simulink model "ode_engine_sim"  (R2022a)
settings: Solver=VariableStepAuto  StartTime=0.0  StopTime=1  MinStep=1e-3
model workspace (MAT data in the model file):
  A_inj = 0.0001076
  C_d = 0.7
  L_grain = 0.6
  PCrit = 72.51
  TCrit = 309.57
  ThermoModel.kin.owner = 1
  ThermoModel.kin.id = 3
  ThermoModel.th.owner = 1
  ThermoModel.th.tp_id = 3
  ThermoModel.tr.id = 3
  ThermoModel.tr.th.owner = 1
  ThermoModel.tr.th.tp_id = 3
  ThermoModel.ThermoPhase.owner = 1
  ThermoModel.ThermoPhase.tp_id = 3
  ThermoModel.Kinetics.owner = 1
  ThermoModel.Kinetics.id = 3
  ThermoModel.Transport.id = 3
  ThermoModel.Transport.th.owner = 1
  ThermoModel.Transport.th.tp_id = 3
  V_tank = 0.0235
  a = 0.397
  inital_cc_pressure = 101325
  inital_run_tank_temperature = 293.3
  m_reg = 1
  n = 0.367
  r_initial = 50
  rhoCrit = 452
  rho_f = 1100
  throat_diam = 0.039385
settings Model: Creator=Artem Sotnikov  LastModifiedBy=Artem Sotnikov
settings SolverCC: MaxConsecutiveMinStep=auto  ShapePreserveControl=EnableAll  ZeroCrossControl=EnableAll  ZeroCrossAlgorithm=Adaptive  EnableFixedStepZeroCrossing=on

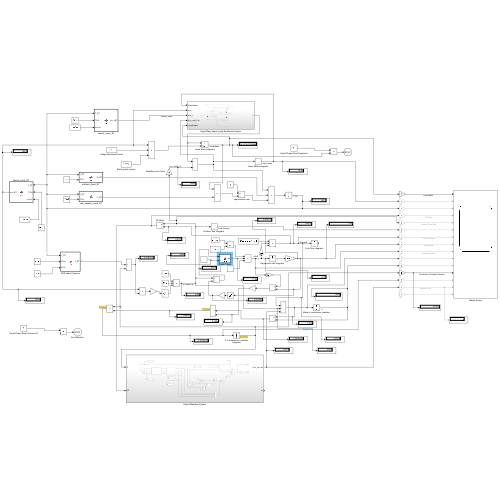
[thumbnail: Simulink's stored preview of the top-level diagram]
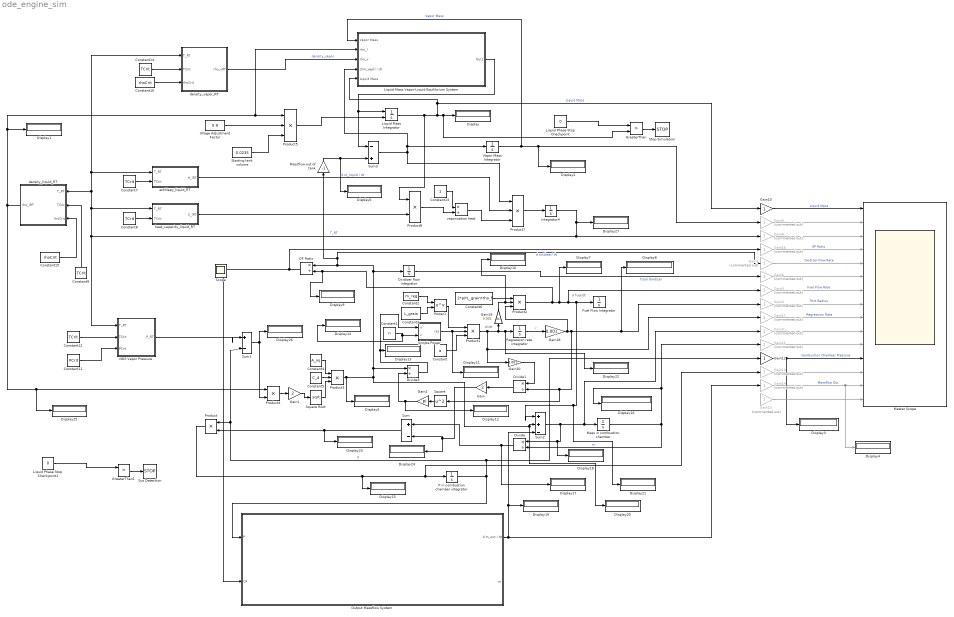
== system ode_engine_sim ==
  note: d fuel/dt
  note: dr/dt
  Constant : Constant  Value=a
  Constant1 : Constant  Value=n
  Constant10 : Constant  Value=rhoCrit
  Constant11 : Constant  Value=PCrit
  Constant{7..9,12,14} (5 alike) : Constant  Value=TCrit
  Constant13 : Constant
  Constant15 : Constant  Value=rhoCrit
  Constant2 : Constant  Value=m_reg
  Constant3 : Constant  Value=L_grain
  Constant4 : Constant  Value=A_inj
  Constant5 : Constant  Value=C_d
  Constant6 : Constant  Value=2*pi*L_grain*rho_f
  Display{,1..27} (28 alike) : Display
  Divide : Product  Inputs=*/
  Divide1 : Product  Inputs=*/
  Divide3 : Product  Inputs=*/
  Fuel Flow Intagrator : Integrator  InitialCondition=1e-6
  Gain : Gain  Gain=2
  Gain1 : Gain  Gain=2
  Gain10 : Gain
  Gain{3..9,11,13..17} (13 alike) : Gain  Commented=on
  Gain12 : Gain
  Gain18 : Gain  Gain=0.001
  Gain19 : Gain  Gain=0.001
  Gain2 : Gain  Gain=pi
  Gain20 : Gain  Gain=0.001
  GreaterThan : RelationalOperator  Operator=>  OutDataTypeStr=boolean  RndMeth=Simplest  InputSameDT=off
  GreaterThan1 : RelationalOperator  Operator=>  OutDataTypeStr=boolean  RndMeth=Simplest  InputSameDT=off
  Integrator4 : Integrator  InitialCondition=inital_run_tank_temperature
  Liquid Mass Integrator : Integrator  InitialConditionSource=external
  Liquid Mass Vapor-Liquid Equilibrium System : Subsystem
  Liquid Phase Stop Checkpoint : Constant  Value=0
  Liquid Phase Stop Checkpoint1 : Constant  Value=0
  Mass in combustion chamber : Integrator  InitialCondition=1e-9
  Massflow out of tank : Gain  Gain=-1
  Master Scope : Scope  NumInputPorts=15
  NOS Vapor Pressure : MATLAB Function  TreatAsAtomicUnit=on
  OF Ratio : Product  Inputs=*/
  Output Massflow System : Subsystem
  Oxidizer flow integrator : Integrator  InitialCondition=1e-6
  P in combustion chamber integrator : Integrator  InitialCondition=inital_cc_pressure  ZeroCross=off
  Power1 : Math  Operator=pow
  Product : Product
  Product{1..3,5,7} (5 alike) : Product  Inputs=3
  Product4 : Product
  Product8 : Product
  Regression rate integrator : Integrator  InitialCondition=r_initial
  Simple Power : MATLAB Function  TreatAsAtomicUnit=on
  Square : Math  Operator=square
  Square Root : Sqrt
  Starting tank volume : Constant  Value=0.0235
  Stop Simulation : Stop
  Sum : Sum  Inputs=|+-  RndMeth=Round
  Sum1 : Sum  Inputs=|+-
  Sum2 : Sum  Inputs=|++-
  Sum3 : Sum  Inputs=-+
  Sus Detection : Stop
  Ullage Adjustment Factor : Constant  Value=0.9
  Vapor Mass Integrator : Integrator  InitialCondition=1e-6
  "density_liquid_RT " : MATLAB Function  TreatAsAtomicUnit=on
  density_vapor_RT : MATLAB Function  TreatAsAtomicUnit=on
  enthlapy_liquid_RT : MATLAB Function  TreatAsAtomicUnit=on
  heat_capacity_liquid_RT : MATLAB Function  TreatAsAtomicUnit=on
  vaporization heat : Product  Inputs=*/
  Scope : Scope
  wires:
  P in combustion chamber integrator/1 -> Gain12/1, Product/1, Sum1/2, Output Massflow System/1(P)  "P"
  Sum/1 -> Display23/1, Product/2
  Mass in combustion chamber/1 -> Display16/1, Gain11/1, Divide/2  "m"
  Product/1 -> Display15/1, Gain13/1, P in combustion chamber integrator/1
  Product1/1 -> Display22/1, Regression rate integrator/1, Gain19/1, Gain17/1, Gain20/1
  Regression rate integrator/1 -> Gain18/1  "r"
  Divide1/1 -> Gain/1
  Power1/1 -> Product1/1
  Constant/1 -> Product1/3
  Constant1/1 -> Simple Power/2(v), Display14/1
  Constant2/1 -> Power1/1
  Constant3/1 -> Power1/2
  Constant5/1 -> Product3/2
  Constant4/1 -> Product3/1
  Square Root/1 -> Product3/3
  Product3/1 -> Display5/1, Display20/1, Sum2/2, Massflow out of tank/1, Gain7/1, OF Ratio/1, Oxidizer flow integrator/1, Divide3/1  "d oxidizer/ dt"
  Gain1/1 -> Square Root/1
  NOS Vapor Pressure/1(P_RT) -> Sum1/1
  Product4/1 -> Gain1/1
  Sum1/1 -> Product4/2, Display26/1
  "density_liquid_RT "/1(rho_lRT) -> Display1/1, Product5/1, Liquid Mass Vapor-Liquid Equilibrium System/2(rho_l), Display25/1, Product4/1
  Square/1 -> Gain2/1
  Gain2/1 -> Display12/1, Divide3/2
  Product2/1 -> Display9/1, OF Ratio/2, Display7/1, Display21/1, Sum2/1, Fuel Flow Intagrator/1, Gain5/1
  Constant6/1 -> Product2/1
  Integrator4/1 -> Display27/1, NOS Vapor Pressure/1(T_RT), enthlapy_liquid_RT/1(T_RT), density_vapor_RT/1(T_RT), "density_liquid_RT "/1(T_RT), heat_capacity_liquid_RT/1(T_RT), Gain8/1  "T_RT"
  Product7/1 -> Integrator4/1
  enthlapy_liquid_RT/1(H_lRT) -> Product7/2
  Constant13/1 -> vaporization heat/1
  Product8/1 -> vaporization heat/2
  heat_capacity_liquid_RT/1(C_lRT) -> Product8/2
  vaporization heat/1 -> Product7/3
  Massflow out of tank/1 -> Display6/1, Sum3/2  "d m_liquid / dt"
  Sum3/1 -> Vapor Mass Integrator/1, Liquid Mass Vapor-Liquid Equilibrium System/4(d(m_vapl) / dt), Product7/1
  Vapor Mass Integrator/1 -> Liquid Mass Vapor-Liquid Equilibrium System/1(Vapor Mass), Display2/1, Gain9/1  "Vapor Mass"
  OF Ratio/1 -> Gain16/1, Output Massflow System/2(OF)
  Output Massflow System/1(d m_out / dt) -> Display19/1, Sum2/3, Gain14/1
  Liquid Mass Vapor-Liquid Equilibrium System/1(Out1) -> Sum3/1, Liquid Mass Integrator/1
  Liquid Mass Integrator/1 -> Product8/1, Display/1, GreaterThan/2, Liquid Mass Vapor-Liquid Equilibrium System/5(Liquid Mass), Gain10/1  "Liquid Mass"
  Oxidizer flow integrator/1 -> Gain6/1  "Total Oxidizer"
  Gain3/1 -> Master Scope/10
  Gain11/1 -> Master Scope/11
  Gain4/1 -> Master Scope/8  "Port Radius"
  Gain5/1 -> Master Scope/7  "Fuel Flow Rate"
  Gain7/1 -> Master Scope/5  "Oxidizer Flow Rate"
  Gain8/1 -> Master Scope/3
  Gain9/1 -> Master Scope/2
  Gain10/1 -> Master Scope/1  "Liquid Mass"
  Gain12/1 -> Display3/1, Master Scope/12  "Combustion Chamber Pressure"
  Gain13/1 -> Master Scope/13
  Gain14/1 -> Display4/1, Master Scope/14  "Massflow Out"
  Gain15/1 -> Master Scope/15
  Gain16/1 -> Master Scope/4  "OF Ratio"
  Gain17/1 -> Master Scope/9  "Regression Rate"
  density_vapor_RT/1(rho_vRT) -> Liquid Mass Vapor-Liquid Equilibrium System/3(rho_v)  "density_vapor"
  Constant7/1 -> enthlapy_liquid_RT/2(TCrit)
  Constant8/1 -> heat_capacity_liquid_RT/2(TCrit)
  Constant9/1 -> "density_liquid_RT "/2(TCrit)
  Constant10/1 -> density_vapor_RT/3(rhoCrit)
  Constant11/1 -> NOS Vapor Pressure/3(PCrit)
  Constant12/1 -> NOS Vapor Pressure/2(TCrit)
  Constant14/1 -> density_vapor_RT/2(TCrit)
  Constant15/1 -> "density_liquid_RT "/3(rhoCrit)
  Gain6/1 -> Master Scope/6
  Starting tank volume/1 -> Product5/3
  Product5/1 -> Liquid Mass Integrator/2
  Ullage Adjustment Factor/1 -> Product5/2
  GreaterThan/1 -> Stop Simulation/1
  Liquid Phase Stop Checkpoint/1 -> GreaterThan/1
  Divide/1 -> Display17/1, Sum/1
  Gain/1 -> Display24/1, Sum/2
  Gain18/1 -> Divide1/2, Square/1, Display8/1, Gain4/1, Product2/3
  Divide3/1 -> Simple Power/1(u), Display13/1
  Simple Power/1(res) -> Display11/1, Product1/2
  Gain19/1 -> Display10/1, Product2/2
  Gain20/1 -> Divide1/1
  Sum2/1 -> Gain3/1, Mass in combustion chamber/1, Display18/1, Divide/1
  Liquid Phase Stop Checkpoint1/1 -> GreaterThan1/1
  GreaterThan1/1 -> Sus Detection/1

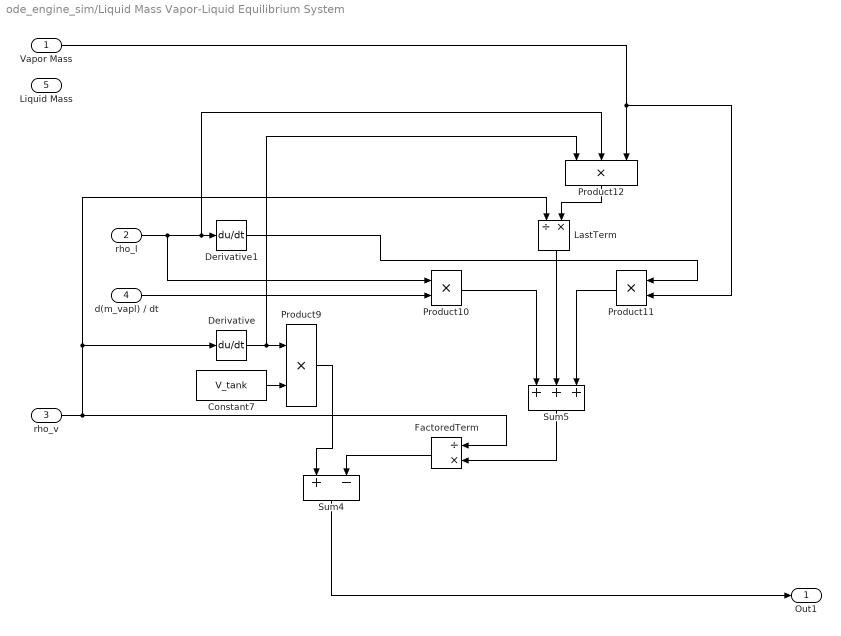
== system ode_engine_sim/Liquid Mass Vapor-Liquid Equilibrium System ==
  Vapor Mass : Inport
  rho_l : Inport  Port=2
  rho_v : Inport  Port=3
  d(m_vapl) / dt : Inport  Port=4
  Liquid Mass : Inport  Port=5
  Constant7 : Constant  Value=V_tank
  Derivative : Derivative
  Derivative1 : Derivative
  FactoredTerm : Product  Inputs=/*
  LastTerm : Product  Inputs=/*
  Product10 : Product
  Product11 : Product
  Product12 : Product  Inputs=3
  Product9 : Product
  Sum4 : Sum  Inputs=+-
  Sum5 : Sum  Inputs=+++
  Out1 : Outport
  wires:
  Product9/1 -> Sum4/1
  Derivative/1 -> Product9/1, Product12/1
  rho_v/1 -> Derivative/1, LastTerm/1, FactoredTerm/1
  Product10/1 -> Sum5/1
  Derivative1/1 -> Product11/1
  LastTerm/1 -> Sum5/2
  Product11/1 -> Sum5/3
  rho_l/1 -> Product10/1, Product12/2, Derivative1/1
  Product12/1 -> LastTerm/2
  Sum5/1 -> FactoredTerm/2
  Constant7/1 -> Product9/2
  FactoredTerm/1 -> Sum4/2
  Sum4/1 -> Out1/1
  d(m_vapl) / dt/1 -> Product10/2
  Vapor Mass/1 -> Product11/2, Product12/3

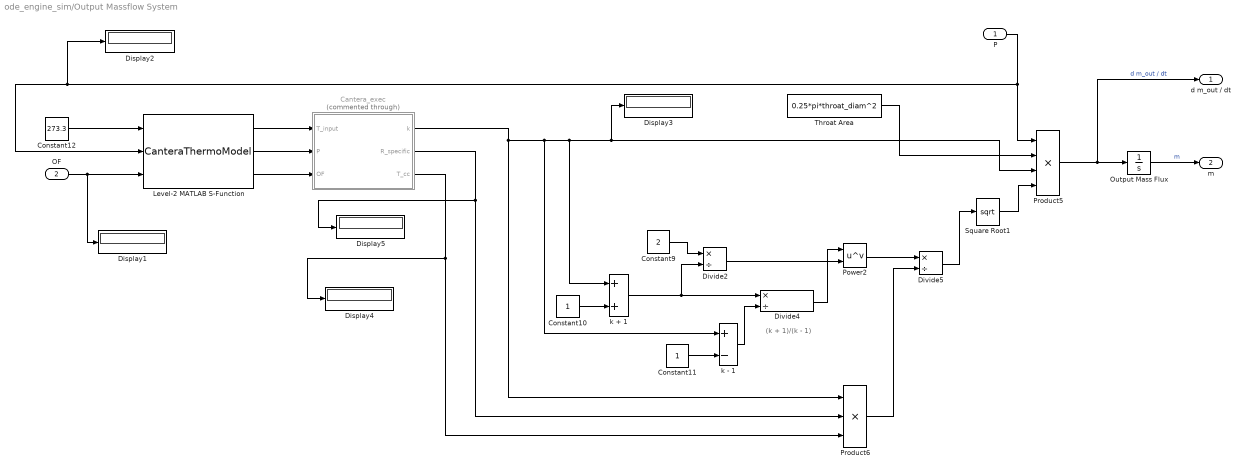
== system ode_engine_sim/Output Massflow System ==
  note: (k + 1)/(k - 1)
  P : Inport
  OF : Inport  Port=2
  Cantera_exec : MATLAB Function  Commented=through  TreatAsAtomicUnit=on
  Constant10 : Constant
  Constant11 : Constant
  Constant12 : Constant  Value=273.3
  Constant9 : Constant  Value=2
  Display{1..5} (5 alike) : Display
  Divide2 : Product  Inputs=*/
  Divide4 : Product  Inputs=*/
  Divide5 : Product  Inputs=*/
  Level-2 MATLAB S-Function : M-S-Function  FunctionName=CanteraThermoModel
  Output Mass Flux : Integrator  InitialCondition=1e-6
  Power2 : Math  Operator=pow
  Product5 : Product  Inputs=4
  Product6 : Product  Inputs=3
  Square Root1 : Sqrt
  Throat Area : Constant  Value=0.25*pi*throat_diam^2
  k + 1 : Sum
  k - 1 : Sum  Inputs=+-
  d m_out / dt : Outport
  m : Outport  Port=2
  wires:
  Divide5/1 -> Square Root1/1
  Product6/1 -> Divide5/2
  k + 1/1 -> Divide4/1, Divide2/2
  Power2/1 -> Divide5/1
  Cantera_exec/1(k) -> Product6/1, Display3/1, Product5/3, k + 1/1, k - 1/1
  Product5/1 -> d m_out / dt/1, Output Mass Flux/1  "d m_out / dt"
  Cantera_exec/3(T_cc) -> Display4/1, Product6/3
  Square Root1/1 -> Product5/4
  Constant9/1 -> Divide2/1
  Cantera_exec/2(R_specific) -> Display5/1, Product6/2
  Output Mass Flux/1 -> m/1  "m"
  Divide2/1 -> Power2/2
  Constant11/1 -> k - 1/2
  Throat Area/1 -> Product5/2
  P/1 -> Display2/1, Level-2 MATLAB S-Function/2, Product5/1
  Constant12/1 -> Level-2 MATLAB S-Function/1
  k - 1/1 -> Divide4/2
  Divide4/1 -> Power2/1
  Constant10/1 -> k + 1/2
  OF/1 -> Display1/1, Level-2 MATLAB S-Function/3
  Level-2 MATLAB S-Function/1 -> Cantera_exec/1(T_input)
  Level-2 MATLAB S-Function/2 -> Cantera_exec/2(P)
  Level-2 MATLAB S-Function/3 -> Cantera_exec/3(OF)

== matlab function ode_engine_sim/Simple Power ==
  data: u input; v input; res output
function res = cpow(u, v)

disp(u)
if u < 0
    print('Alert!')
end

res = u^v;

== matlab function ode_engine_sim/NOS Vapor Pressure ==
  data: T_RT input; TCrit input; P_RT output; PCrit input
function P_RT = fcn(T_RT, TCrit, PCrit)

p = [1.0, 1.5, 2.5, 5.0];
b = [-6.71893, 1.35966, -1.3779, -4.051];

Tr = T_RT / TCrit;
Tr_minus_one_vP = 1.0 - Tr;
acc_vP = 0.0;

for idx = [1,2,3,4]
    acc_vP = acc_vP + b(idx) * Tr_minus_one_vP^p(idx);
end

P_RT_bar = PCrit * exp((acc_vP / Tr));
P_RT = P_RT_bar * 100000; % conversion bar -> Pa

== matlab function ode_engine_sim/Output Massflow System/Cantera_exec ==
  data: k output; R_specific output; T_input input; T_cc output; P input; OF input
function [k, R_specific, T_cc] = fcn(T_input, P, OF)

if isempty(ThermoModel)

end

coder.extrinsic('set');
set(ThermoModel, 'T', T_input, 'P', P, 'Y', sprintf("N2O:%f.3, C4H6:1", OF));

coder.extrinsic('temperature');
coder.extrinsic('equilibrate');
coder.extrinsic('meanMolecularWeight');
coder.extrinsic('cp_mass');
coder.extrinsic('cv_mass');

equilibrate(ThermoModel, 'HP');


T_cc = zeros(1);
k = zeros(1);
R_specific = zeros(1);


T_cc = temperature(ThermoModel);
k = cp_mass(ThermoModel)/cv_mass(ThermoModel);
R_specific = 8314 / meanMolecularWeight(ThermoModel);

== matlab function ode_engine_sim/heat_capacity_liquid_RT ==
  data: T_RT input; C_lRT output; TCrit input
function C_lRT = fcn(T_RT, TCrit)

b = [2.49973, 0.023454, -3.80136, 13.0945, -14.518];

Tr_C = T_RT / TCrit;
Tr_C_minus_one = 1.0 - Tr_C;
acc = 1.0 + b(1) / Tr_C_minus_one;


for idx = [1,2,3,4]
    acc = acc + b(idx) * Tr_C_minus_one^idx;
end

result = b(1) * acc * 1000.0; % convert from KJ to J */

C_lRT = result;

== matlab function ode_engine_sim/enthlapy_liquid_RT ==
  data: T_RT input; H_lRT output; TCrit input
function H_lRT = fcn(T_RT, TCrit)
bL = [-200.0, 116.043, -917.225, 794.779, -589.587];
bV = [-200.0, 440.055, -459.701, 434.081, -485.338];

Tr_H = T_RT / TCrit;
Tr_H_minus_one = 1.0 - Tr_H;
acc_L = bL(1);
acc_V = bV(1);


for idx = [1,2,3,4,5]
    acc_L = acc_L + bL(idx) * Tr_H_minus_one^(idx / 3.0); 
    acc_V = acc_V + bV(idx) * Tr_H_minus_one^(idx / 3.0); 
end

result = (acc_V - acc_L) * 1000.0;

H_lRT = result;

== matlab function ode_engine_sim/density_liquid_RT  ==
  data: T_RT input; rho_lRT output; TCrit input; rhoCrit input
function rho_lRT = fcn(T_RT, TCrit, rhoCrit)

b = [1.72328, -0.8395, 0.5106, -0.10412];

Tr_l = T_RT / TCrit;
Tr_l_minus_one = 1.0 - Tr_l;
acc_l = 0.0;

for idx = [1,2,3,4]
    acc_l = acc_l + b(idx)* Tr_l_minus_one^(idx/3.0);
end

rho_lRT = rhoCrit * exp(acc_l);

== matlab function ode_engine_sim/density_vapor_RT ==
  data: T_RT input; TCrit input; rho_vRT output; rhoCrit input
function rho_vRT = fcn(T_RT, TCrit, rhoCrit)

b = [-1.009, -6.28792, 7.50332, -7.90463, 0.629427];

Tr_v = T_RT / TCrit;
Tr_v_minus_one = 1.0 - Tr_v;
acc_v = 0.0;

for idx = [1,2,3,4,5]
    acc_v = acc_v + b(idx) * Tr_v_minus_one^(idx/3.0);
end


rho_vRT = rhoCrit * exp(acc_v);
